simulink model "model_T_PSH_IEEE39"  (R2020b)
settings: Solver=ode3  StartTime=0.0  StopTime=300  FixedStep=Ts  RelTol=1e-3
PostLoadFcn:
  | IEEE39BusLineLength;
  | vNomHV = 345E3;fNom=60;load('Dynamicload.mat');
InitFcn:
  | IEEE39BusLineLength;
  | vNomHV = 345E3;fNom=60;load('Dynamicload.mat');
values from neighbouring files (symbols this model uses):
  At = 1.48    [MAIN_T_PSH_IEEE39.m]
  Dturb = 0.3    [MAIN_T_PSH_IEEE39.m]
  fix_mode = 1    [MAIN_T_PSH_IEEE39.m]
  Gmax = 1    [MAIN_T_PSH_IEEE39.m]
  Gmin = 0    [MAIN_T_PSH_IEEE39.m]
  Hdam = 1    [MAIN_T_PSH_IEEE39.m]
  Kd = 1    [MAIN_T_PSH_IEEE39.m]    (also in plots_T_PSH_IEEE39.m)
  max_delay_gen2pump = 20    [MAIN_T_PSH_IEEE39.m]
  max_delay_pump2hsc = 30    [MAIN_T_PSH_IEEE39.m]
  pgen_pump = Kd*Pref    (= 0.9)    [MAIN_T_PSH_IEEE39.m]
  pgen_turb = (1-Kd)*Pref    (= 0)    [MAIN_T_PSH_IEEE39.m]
  pgen_turb_gen2pump = (1-kd_gen2pump)*Pref    (= 0)    [MAIN_T_PSH_IEEE39.m]
  pgen_turb_hsc2gen = (1-kd_hsc2gen)*Pref    (= 0.36)    [MAIN_T_PSH_IEEE39.m]
  pgen_turb_pump2hsc = (1-kd_pump2hsc)*Pref    (= 0.36)    [MAIN_T_PSH_IEEE39.m]
  Pref = 0.9    [MAIN_T_PSH_IEEE39.m]    (also in MAIN_VS_PSH.m = 1)
  qNL = 0.1    [MAIN_T_PSH_IEEE39.m]
  R = 0.04    [MAIN_T_PSH_IEEE39.m]
  r = 0.31    [MAIN_T_PSH_IEEE39.m]
  Rp = 0.05    [IEEE39BusLineLength.m]
  Sn = 320E6    (= 320000000)    [MAIN_T_PSH_IEEE39.m]
  t_gen2pump = 10    [MAIN_T_PSH_IEEE39.m]
  t_hsc2gen = 150    [MAIN_T_PSH_IEEE39.m]
  t_pump2hsc = 35    [MAIN_T_PSH_IEEE39.m]
  t_sw_off = 220    [MAIN_FS_PSH_IEEE39.m]    (also in MAIN_T_PSH_IEEE39.m; MAIN_VS_PSH.m = 45)
  t_sw_on = 130    [MAIN_FS_PSH_IEEE39.m]    (also in MAIN_T_PSH_IEEE39.m; MAIN_VS_PSH.m = 35)
  Tf = 0.05    [MAIN_T_PSH_IEEE39.m]
  Tg = 0.5    [MAIN_T_PSH_IEEE39.m]
  TL_10_11_len = 14    [IEEE39BusLineLength.m]
  TL_10_13_len = 14    [IEEE39BusLineLength.m]
  TL_13_14_len = 32    [IEEE39BusLineLength.m]
  TL_14_15_len = 70    [IEEE39BusLineLength.m]
  TL_15_16_len = 31.5    [IEEE39BusLineLength.m]
  TL_16_17_len = 26    [IEEE39BusLineLength.m]
  TL_16_19_len = 61    [IEEE39BusLineLength.m]
  TL_16_21_len = 46    [IEEE39BusLineLength.m]
  TL_16_24_len = 15    [IEEE39BusLineLength.m]
  TL_17_18_len = 26    [IEEE39BusLineLength.m]
  TL_17_27_len = 59    [IEEE39BusLineLength.m]
  TL_1_2_len = 134    [IEEE39BusLineLength.m]
  TL_1_39_len = 105    [IEEE39BusLineLength.m]
  TL_21_22_len = 47    [IEEE39BusLineLength.m]
  TL_22_23_len = 33    [IEEE39BusLineLength.m]
  TL_24_23_len = 88    [IEEE39BusLineLength.m]
  TL_25_26_len = 101    [IEEE39BusLineLength.m]
  TL_26_27_len = 46.5    [IEEE39BusLineLength.m]
  TL_26_28_len = 151    [IEEE39BusLineLength.m]
  TL_26_29_len = 200    [IEEE39BusLineLength.m]
  TL_28_29_len = 48    [IEEE39BusLineLength.m]
  TL_2_25_len = 28    [IEEE39BusLineLength.m]
  TL_2_2_len = 49    [IEEE39BusLineLength.m]
  TL_3_18_len = 42    [IEEE39BusLineLength.m]
  TL_3_4_len = 53    [IEEE39BusLineLength.m]
  TL_4_14_len = 33    [IEEE39BusLineLength.m]
  TL_4_5_len = 32.5    [IEEE39BusLineLength.m]
  TL_5_6_len = 14    [IEEE39BusLineLength.m]
  TL_5_8_len = 32    [IEEE39BusLineLength.m]
  TL_6_11_len = 26.5    [IEEE39BusLineLength.m]
  TL_6_7_len = 25.5    [IEEE39BusLineLength.m]
  TL_7_8_len = 15    [IEEE39BusLineLength.m]
  TL_8_9_len = 93    [IEEE39BusLineLength.m]
  TL_9_39_len = 136    [IEEE39BusLineLength.m]
  Tr = 6.88    [MAIN_T_PSH_IEEE39.m]
  Ts = 25e-6    (= 2.5e-05)    [MAIN_FS_PSH_IEEE39.m]    (also in MAIN_T_PSH_IEEE39.m; MAIN_VS_PSH.m = 1e-07)
  Velm = 0.05    [MAIN_T_PSH_IEEE39.m]
  Vn = 18000    [MAIN_T_PSH_IEEE39.m]
undefined symbols (not defined in the file or in its folder): D1, Delta, load15, load16, load18, load20, load21, load23, load24, load25, load26, load27, load28, load29, load3, load39, load4, load7, load8
libraries: powerlib x216, sps_avr x10, simulink_extras x7, powerlib_meascontrol x5, simulink x1
(part 6 of 9)

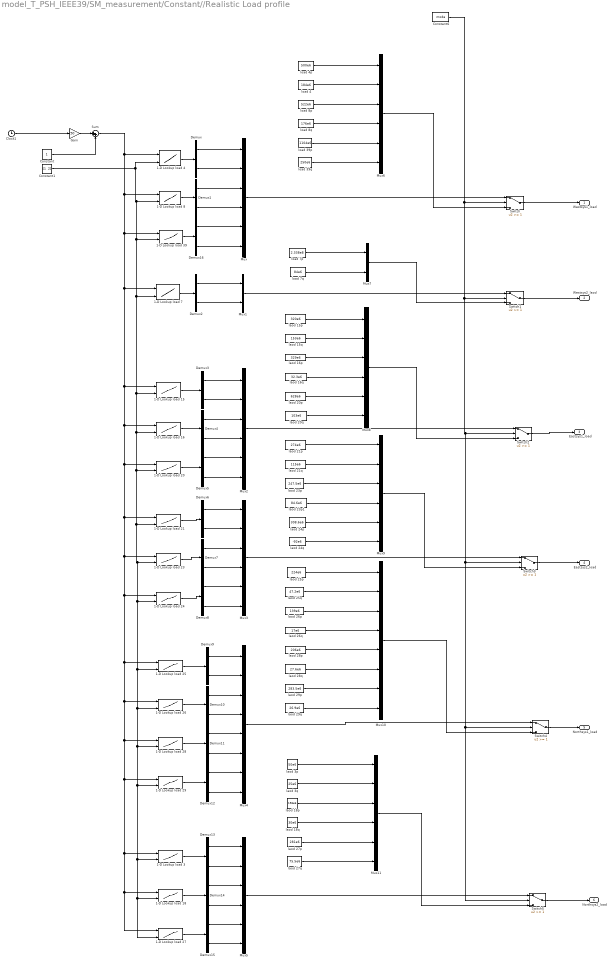
== system model_T_PSH_IEEE39/SM_measurement/Constant//Realistic Load profile ==
  1-D Lookup load 15 : Lookup_n-D  BreakpointsForDimension1=[1:18000]  BreakpointsForDimension2=[1 2]  Table=load15  InterpMethod=Flat  ExtrapMethod=Cubic spline  DiagnosticForOutOfRangeInput=Error  InternalRulePriority=Speed  RndMeth=Simplest  InputSameDT=on
      settings: InputPortMap=u0,u1
  1-D Lookup load 16 : Lookup_n-D  BreakpointsForDimension1=[1:18000]  BreakpointsForDimension2=[1 2]  Table=load16  InterpMethod=Flat  ExtrapMethod=Cubic spline  DiagnosticForOutOfRangeInput=Error  InternalRulePriority=Speed  RndMeth=Simplest  InputSameDT=on
      settings: InputPortMap=u0,u1
  1-D Lookup load 18 : Lookup_n-D  BreakpointsForDimension1=[1:18000]  BreakpointsForDimension2=[1 2]  Table=load18  InterpMethod=Flat  ExtrapMethod=Cubic spline  DiagnosticForOutOfRangeInput=Error  InternalRulePriority=Speed  RndMeth=Simplest  InputSameDT=on
      settings: InputPortMap=u0,u1
  1-D Lookup load 20 : Lookup_n-D  BreakpointsForDimension1=[1:18000]  BreakpointsForDimension2=[1 2]  Table=load20  InterpMethod=Flat  ExtrapMethod=Cubic spline  DiagnosticForOutOfRangeInput=Error  InternalRulePriority=Speed  RndMeth=Simplest  InputSameDT=on
      settings: InputPortMap=u0,u1
  1-D Lookup load 21 : Lookup_n-D  BreakpointsForDimension1=[1:18000]  BreakpointsForDimension2=[1 2]  Table=load21  InterpMethod=Flat  ExtrapMethod=Cubic spline  DiagnosticForOutOfRangeInput=Error  InternalRulePriority=Speed  RndMeth=Simplest  InputSameDT=on
      settings: InputPortMap=u0,u1
  1-D Lookup load 23 : Lookup_n-D  BreakpointsForDimension1=[1:18000]  BreakpointsForDimension2=[1 2]  Table=load23  InterpMethod=Flat  ExtrapMethod=Cubic spline  DiagnosticForOutOfRangeInput=Error  InternalRulePriority=Speed  RndMeth=Simplest  InputSameDT=on
      settings: InputPortMap=u0,u1
  1-D Lookup load 24 : Lookup_n-D  BreakpointsForDimension1=[1:18000]  BreakpointsForDimension2=[1 2]  Table=load24  InterpMethod=Flat  ExtrapMethod=Cubic spline  DiagnosticForOutOfRangeInput=Error  InternalRulePriority=Speed  RndMeth=Simplest  InputSameDT=on
      settings: InputPortMap=u0,u1
  1-D Lookup load 25 : Lookup_n-D  BreakpointsForDimension1=[1:18000]  BreakpointsForDimension2=[1 2]  Table=load25  InterpMethod=Flat  ExtrapMethod=Cubic spline  DiagnosticForOutOfRangeInput=Error  InternalRulePriority=Speed  RndMeth=Simplest  InputSameDT=on
      settings: InputPortMap=u0,u1
  1-D Lookup load 26 : Lookup_n-D  BreakpointsForDimension1=[1:18000]  BreakpointsForDimension2=[1 2]  Table=load26  InterpMethod=Flat  ExtrapMethod=Cubic spline  DiagnosticForOutOfRangeInput=Error  InternalRulePriority=Speed  RndMeth=Simplest  InputSameDT=on
      settings: InputPortMap=u0,u1
  1-D Lookup load 27 : Lookup_n-D  BreakpointsForDimension1=[1:18000]  BreakpointsForDimension2=[1 2]  Table=load27  InterpMethod=Flat  ExtrapMethod=Cubic spline  DiagnosticForOutOfRangeInput=Error  InternalRulePriority=Speed  RndMeth=Simplest  InputSameDT=on
      settings: InputPortMap=u0,u1
  1-D Lookup load 28 : Lookup_n-D  BreakpointsForDimension1=[1:18000]  BreakpointsForDimension2=[1 2]  Table=load28  InterpMethod=Flat  ExtrapMethod=Cubic spline  DiagnosticForOutOfRangeInput=Error  InternalRulePriority=Speed  RndMeth=Simplest  InputSameDT=on
      settings: InputPortMap=u0,u1
  1-D Lookup load 29 : Lookup_n-D  BreakpointsForDimension1=[1:18000]  BreakpointsForDimension2=[1 2]  Table=load29  InterpMethod=Flat  ExtrapMethod=Cubic spline  DiagnosticForOutOfRangeInput=Error  InternalRulePriority=Speed  RndMeth=Simplest  InputSameDT=on
      settings: InputPortMap=u0,u1
  1-D Lookup load 3 : Lookup_n-D  BreakpointsForDimension1=[1:18000]  BreakpointsForDimension2=[1 2]  Table=load3  InterpMethod=Flat  ExtrapMethod=Cubic spline  DiagnosticForOutOfRangeInput=Error  InternalRulePriority=Speed  RndMeth=Simplest  InputSameDT=on
      settings: InputPortMap=u0,u1
  1-D Lookup load 39 : Lookup_n-D  BreakpointsForDimension1=[1:18000]  BreakpointsForDimension2=[1 2]  Table=load39  InterpMethod=Flat  ExtrapMethod=Cubic spline  DiagnosticForOutOfRangeInput=Error  InternalRulePriority=Speed  RndMeth=Simplest  InputSameDT=on
      settings: InputPortMap=u0,u1
  1-D Lookup load 4 : Lookup_n-D  BreakpointsForDimension1=[1:18000]  BreakpointsForDimension2=[1 2]  Table=load4  InterpMethod=Flat  ExtrapMethod=Cubic spline  DiagnosticForOutOfRangeInput=Error  InternalRulePriority=Speed  RndMeth=Simplest  InputSameDT=on
      settings: InputPortMap=u0,u1
  1-D Lookup load 7 : Lookup_n-D  BreakpointsForDimension1=[1:18000]  BreakpointsForDimension2=[1 2]  Table=load7  InterpMethod=Flat  ExtrapMethod=Cubic spline  DiagnosticForOutOfRangeInput=Error  InternalRulePriority=Speed  RndMeth=Simplest  InputSameDT=on
      settings: InputPortMap=u0,u1
  1-D Lookup load 8 : Lookup_n-D  BreakpointsForDimension1=[1:18000]  BreakpointsForDimension2=[1 2]  Table=load8  InterpMethod=Flat  ExtrapMethod=Cubic spline  DiagnosticForOutOfRangeInput=Error  InternalRulePriority=Speed  RndMeth=Simplest  InputSameDT=on
      settings: InputPortMap=u0,u1
  Clock1 : Clock
  Constant : Constant  SampleTime=20e-3
  Constant1 : Constant  Value="[1  2]"  VectorParams1D=off  SampleTime=20e-3
  Constant6 : Constant  Value=mode
  Demux{,1..16} (17 alike) : Demux  Outputs=2
  Gain : Gain  Gain=50
  Mux{,2..3,5..6,8..9,11} (8 alike) : Mux  Inputs=6
  Mux1 : Mux  Inputs=2
  Mux10 : Mux  Inputs=8
  Mux4 : Mux  Inputs=8
  Mux7 : Mux  Inputs=2
  Sum : Sum  Inputs=|++
  Switch{,1..5} (6 alike) : Switch  Threshold=1
  laod 15p : Constant  Value=320e6  VectorParams1D=off  SampleTime=20e-3
  laod 15q : Constant  Value=153e6  VectorParams1D=off  SampleTime=20e-3
  laod 16p : Constant  Value=329e6  VectorParams1D=off  SampleTime=20e-3
  laod 16q : Constant  Value=32.3e6  VectorParams1D=off  SampleTime=20e-3
  laod 18p : Constant  Value=158e6  VectorParams1D=off  SampleTime=20e-3
  laod 18q : Constant  Value=30e6  VectorParams1D=off  SampleTime=20e-3
  laod 20p : Constant  Value=628e6  VectorParams1D=off  SampleTime=20e-3
  laod 20q : Constant  Value=103e6  VectorParams1D=off  SampleTime=20e-3
  laod 21p : Constant  Value=274e6  VectorParams1D=off  SampleTime=20e-3
  laod 21q : Constant  Value=115e6  VectorParams1D=off  SampleTime=20e-3
  laod 23p : Constant  Value=247.5e6  VectorParams1D=off  SampleTime=20e-3
  laod 23p1 : Constant  Value=84.6e6  VectorParams1D=off  SampleTime=20e-3
  laod 24p : Constant  Value=308.6e6  SampleTime=20e-3
  laod 24q : Constant  Value=-92e6  VectorParams1D=off  SampleTime=20e-3
  laod 25p : Constant  Value=224e6  VectorParams1D=off  SampleTime=20e-3
  laod 25q : Constant  Value=47.2e6  VectorParams1D=off  SampleTime=20e-3
  laod 26p : Constant  Value=139e6  VectorParams1D=off  SampleTime=20e-3
  laod 26q : Constant  Value=17e6  VectorParams1D=off  SampleTime=20e-3
  laod 27p : Constant  Value=281e6  VectorParams1D=off  SampleTime=20e-3
  laod 27q : Constant  Value=75.5e6  VectorParams1D=off  SampleTime=20e-3
  laod 28p : Constant  Value=206e6  VectorParams1D=off  SampleTime=20e-3
  laod 28q : Constant  Value=27.6e6  VectorParams1D=off  SampleTime=20e-3
  laod 29p : Constant  Value=283.5e6  VectorParams1D=off  SampleTime=20e-3
  laod 29q : Constant  Value=26.9e6  VectorParams1D=off  SampleTime=20e-3
  laod 3p : Constant  Value=50e6  VectorParams1D=off  SampleTime=20e-3
  laod 3q : Constant  Value=25e6  VectorParams1D=off  SampleTime=20e-3
  load 39p : Constant  Value=1104e6  VectorParams1D=off  SampleTime=20e-3
  load 39q : Constant  Value=250e6  VectorParams1D=off  SampleTime=20e-3
  load 4 : Constant  Value=184e6  VectorParams1D=off  SampleTime=20e-3
  load 4p : Constant  Value=500e6  VectorParams1D=off  SampleTime=20e-3
  load 7p : Constant  Value=2.338e8  VectorParams1D=off  SampleTime=20e-3
  load 7q : Constant  Value=84e6  VectorParams1D=off  SampleTime=20e-3
  load 8p : Constant  Value=522e6  VectorParams1D=off  SampleTime=20e-3
  load 8q : Constant  Value=176e6  VectorParams1D=off  SampleTime=20e-3
  Westsys1_load : Outport
  Westsys2_laod : Outport  Port=2
  Eastsys1_load : Outport  Port=3
  Eastsys2_load : Outport  Port=4
  Northsys1_load : Outport  Port=5
  Northsys2_load : Outport  Port=6
  wires:
  Mux2/1 -> Switch2/1
  Constant/1 -> Sum/2
  Mux/1 -> Switch/1
  Mux1/1 -> Switch1/1
  Mux5/1 -> Switch5/1
  1-D Lookup load 15/1 -> Demux3/1
  Demux2/2 -> Mux1/2
  Demux5/2 -> Mux2/6
  Demux7/2 -> Mux3/4
  Demux10/2 -> Mux4/4
  Sum/1 -> 1-D Lookup load 28/1, 1-D Lookup load 27/1, 1-D Lookup load 18/1, 1-D Lookup load 3/1, 1-D Lookup load 29/1, 1-D Lookup load 26/1, 1-D Lookup load 25/1, 1-D Lookup load 24/1, 1-D Lookup load 23/1, 1-D Lookup load 21/1, 1-D Lookup load 20/1, 1-D Lookup load 16/1, 1-D Lookup load 15/1, 1-D Lookup load 7/1, 1-D Lookup load 39/1, 1-D Lookup load 8/1, 1-D Lookup load 4/1
  1-D Lookup load 4/1 -> Demux/1
  Demux/1 -> Mux/1
  Demux/2 -> Mux/2
  1-D Lookup load 8/1 -> Demux1/1
  Demux1/1 -> Mux/3
  Demux1/2 -> Mux/4
  Demux16/1 -> Mux/5
  Demux16/2 -> Mux/6
  1-D Lookup load 39/1 -> Demux16/1
  1-D Lookup load 7/1 -> Demux2/1
  Demux2/1 -> Mux1/1
  Demux3/1 -> Mux2/1
  Demux3/2 -> Mux2/2
  1-D Lookup load 16/1 -> Demux4/1
  Demux4/1 -> Mux2/3
  Demux4/2 -> Mux2/4
  Demux5/1 -> Mux2/5
  1-D Lookup load 20/1 -> Demux5/1
  Demux6/2 -> Mux3/2
  Demux6/1 -> Mux3/1
  1-D Lookup load 21/1 -> Demux6/1
  Demux7/1 -> Mux3/3
  1-D Lookup load 23/1 -> Demux7/1
  1-D Lookup load 24/1 -> Demux8/1
  Demux8/1 -> Mux3/5
  Demux8/2 -> Mux3/6
  Demux9/2 -> Mux4/2
  Demux9/1 -> Mux4/1
  1-D Lookup load 25/1 -> Demux9/1
  1-D Lookup load 26/1 -> Demux10/1
  Demux10/1 -> Mux4/3
  Demux11/1 -> Mux4/5
  Demux11/2 -> Mux4/6
  1-D Lookup load 28/1 -> Demux11/1
  Demux12/1 -> Mux4/7
  Demux12/2 -> Mux4/8
  1-D Lookup load 29/1 -> Demux12/1
  1-D Lookup load 3/1 -> Demux13/1
  Demux13/1 -> Mux5/1
  Demux13/2 -> Mux5/2
  Constant1/1 -> 1-D Lookup load 7/2, 1-D Lookup load 20/2, 1-D Lookup load 27/2, 1-D Lookup load 18/2, 1-D Lookup load 3/2, 1-D Lookup load 29/2, 1-D Lookup load 28/2, 1-D Lookup load 26/2, 1-D Lookup load 25/2, 1-D Lookup load 24/2, 1-D Lookup load 23/2, 1-D Lookup load 21/2, 1-D Lookup load 16/2, 1-D Lookup load 15/2, 1-D Lookup load 39/2, 1-D Lookup load 8/2, 1-D Lookup load 4/2
  Demux14/1 -> Mux5/3
  Demux14/2 -> Mux5/4
  1-D Lookup load 18/1 -> Demux14/1
  Demux15/1 -> Mux5/5
  Demux15/2 -> Mux5/6
  1-D Lookup load 27/1 -> Demux15/1
  Clock1/1 -> Gain/1
  Gain/1 -> Sum/1
  Mux6/1 -> Switch/3
  load 4p/1 -> Mux6/1
  load 4/1 -> Mux6/2
  load 8p/1 -> Mux6/3
  load 8q/1 -> Mux6/4
  load 39p/1 -> Mux6/5
  load 39q/1 -> Mux6/6
  Constant6/1 -> Switch5/2, Switch4/2, Switch3/2, Switch2/2, Switch1/2, Switch/2
  Switch/1 -> Westsys1_load/1
  Mux7/1 -> Switch1/3
  load 7q/1 -> Mux7/2
  load 7p/1 -> Mux7/1
  Switch1/1 -> Westsys2_laod/1
  Switch2/1 -> Eastsys1_load/1
  laod 20q/1 -> Mux8/6
  laod 15p/1 -> Mux8/1
  laod 15q/1 -> Mux8/2
  laod 16p/1 -> Mux8/3
  laod 16q/1 -> Mux8/4
  laod 20p/1 -> Mux8/5
  Mux8/1 -> Switch2/3
  Switch3/1 -> Eastsys2_load/1
  Mux3/1 -> Switch3/1
  laod 23p1/1 -> Mux9/4
  laod 21q/1 -> Mux9/2
  laod 21p/1 -> Mux9/1
  laod 23p/1 -> Mux9/3
  laod 24p/1 -> Mux9/5
  laod 24q/1 -> Mux9/6
  Mux9/1 -> Switch3/3
  Mux10/1 -> Switch4/3
  laod 26q/1 -> Mux10/4
  laod 25q/1 -> Mux10/2
  laod 25p/1 -> Mux10/1
  laod 26p/1 -> Mux10/3
  laod 28p/1 -> Mux10/5
  laod 28q/1 -> Mux10/6
  laod 29p/1 -> Mux10/7
  laod 29q/1 -> Mux10/8
  Switch4/1 -> Northsys1_load/1
  Mux4/1 -> Switch4/1
  Mux11/1 -> Switch5/3
  laod 3p/1 -> Mux11/1
  laod 3q/1 -> Mux11/2
  laod 18p/1 -> Mux11/3
  laod 18q/1 -> Mux11/4
  laod 27p/1 -> Mux11/5
  laod 27q/1 -> Mux11/6
  Switch5/1 -> Northsys2_load/1

== system model_T_PSH_IEEE39/SM_measurement/GT control ==
  note: 10
  note: 9
  note: 8
  note: 7
  note: 6
  note: 5
  note: 4
  note: 3
  note: 2
  note: 1
  Bus Creator : BusCreator  Inputs=3
  Constant{1..6,8,10,12,14} (10 alike) : Constant
  Mux1 : Mux  Inputs=3
  Mux2 : Mux
  Mux6 : Mux  Inputs=3
  GT_CBs_ctrl : Outport
  wires:
  Constant1/1 -> Mux1/2
  Constant10/1 -> Mux1/1
  Constant12/1 -> Mux2/4
  Constant5/1 -> Mux2/3
  Constant2/1 -> Mux2/2
  Constant3/1 -> Mux2/1
  Constant4/1 -> Mux6/3
  Constant8/1 -> Mux6/2
  Constant14/1 -> Mux1/3
  Constant6/1 -> Mux6/1
  Bus Creator/1 -> GT_CBs_ctrl/1
  Mux2/1 -> Bus Creator/2  "Eastsystem GT ctrl"
  Mux6/1 -> Bus Creator/1  "Westsystem GT ctrl"
  Mux1/1 -> Bus Creator/3  "Northsystem GT ctrl"

== system model_T_PSH_IEEE39/SS_EastSystem1/Buses current_E ==
  Mux3 : Mux  Inputs=5
  current : Outport
  wires:
  Mux3/1 -> current/1
  [I_bus_14] -> Mux3/1
  [I_L15] -> Mux3/2
  [I_L16] -> Mux3/3
  [I_bus_19] -> Mux3/4
  [I_L20] -> Mux3/5

== system model_T_PSH_IEEE39/SS_EastSystem1/Buses voltages_E ==
  Mux3 : Mux  Inputs=5
  Voltages : Outport
  wires:
  [V_L20] -> Mux3/5
  [V_bus_19] -> Mux3/4
  [V_L16] -> Mux3/3
  [V_L15] -> Mux3/2
  [V_bus_14] -> Mux3/1
  Mux3/1 -> Voltages/1

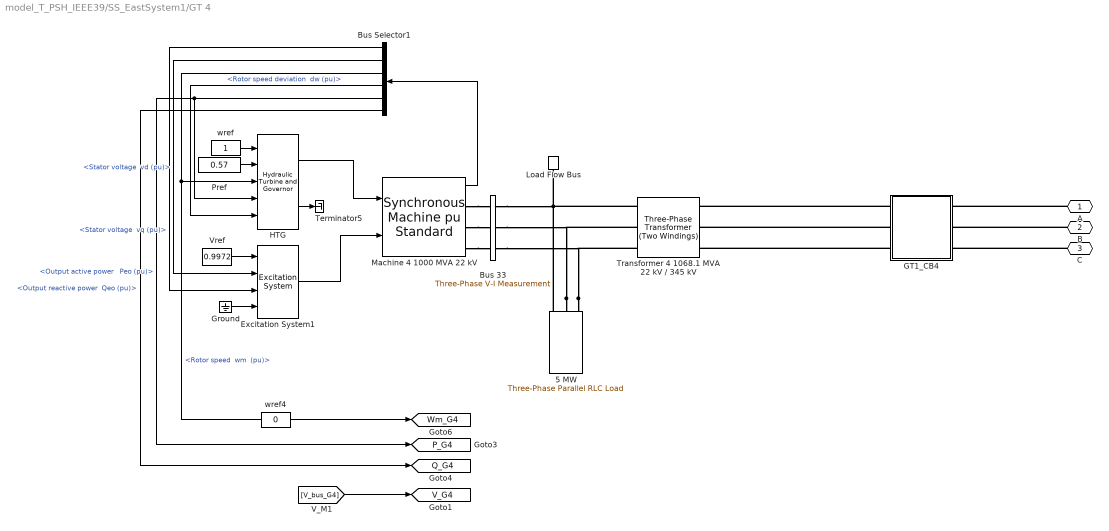
== system model_T_PSH_IEEE39/SS_EastSystem1/GT 4 ==
  5 MW : powerlib/Elements/Three-Phase Parallel RLC Load  LConnTagsString=A|B|C  Configuration=Y (grounded)  NominalVoltage=22e3  Vabc=[1e3 1e3 1e3]  Vabcp=[1e3 1e3 1e3]  NominalFrequency=fNom  UnbalancedPower=off  ActivePower=5e6  InductivePower=0  CapacitivePower=0  Pabc=[10e3 9e3 11e3]  QLabc=[100 90 110]  QCabc=[100 90 110]  Pabcp=[10e3 9e3 11e3]  QLabcp=[100 90 110]  QCabcp=[100 90 110]  Measurements=None  LoadType=constant Z
  Bus Selector1 : BusSelector  OutputSignals="dq0 components.Stator voltage  vq (pu),dq0 components.Stator voltage  vd (pu),Mechanical.Rotor speed  wm  (pu),Mechanical.Rotor speed deviation  dw (pu),Output active power   Peo (pu),Output reactive power  Qeo (pu)"
  Bus 33 : powerlib/Measurements/Three-Phase V-I Measurement  VoltageMeasurement=phase-to-ground  SetLabelV=on  LabelV=V_bus_G4  Vpu=off  VpuLL=off  CurrentMeasurement=no  SetLabelI=on  LabelI=I_bus_G4  Ipu=off  Pbase=100e6  Vbase=16.5e3  OutputType=Complex  PhasorSimulation=off  PSBequivalent=0
  Excitation System1 : sps_avr/Excitation System  tr=20e-3  reg=[ 200, 0.02 ]  exc=[ 1, 0 .19]  tgr=[ 0, 0 ]  damp=[ 0.0012, 1 ]  sat=[ 0, 0 ]  lim=[ 0, 7.32, 0 ]  v0=[0.9972 1.7419]
      settings: SourceProductBaseCode=PS
  GT1_CB4 : Subsystem
  Ground : Ground
  HTG : powerlib/Machines/Hydraulic Turbine and Governor  sm="[ 10/3  0.07 ]"  gate="[  0.01  0.97518  -0.1  0.1 ]"  reg="[ Rp  1.163  0.105  0  0.01  ]"  hyd="[  0  2.67  ]"  dref=0  po=0.57
      settings: SourceProductBaseCode=PS
  Load Flow Bus : powerlib/Measurements/Load Flow Bus  LConnTagsString=a  Phases=single  Connectors=on one side  ID=Bus-33  Vbase=22000  Vref=0.9972  Vangle=0  VLF=0.9972  VLFb=1  VLFc=1  angleLF=-4.252  angleLFb=0  angleLFc=0
      settings: AttributesFormatString=%<ID>\n%<Vbase>V\n%<VLF>pu\n%<angleLF>deg.
  Machine 4 1000 MVA 22 kV : powerlib/Machines/Synchronous Machine pu Standard  PresetModel=No  MechanicalLoad=Mechanical power Pm  ShowDetailedParameters=on  RotorType=Round  Units=per unit standard parameters  MeasurementBus=off  NominalParameters="[ 1000E6  22000   fNom]"  Reactances1="[ 2.403 0.4 0.2 2.367 1.523 0.2 0.03  ]"  Reactances2=[ 0.995, 0.195, 0.155, 0.568, 0.143, 0.16 ]  dAxisTimeConstants=Open-circuit  qAxisTimeConstants=Open-circuit  TimeConstants1=[]  TimeConstants2=[5.69 0.03 1.5 0.04]  TimeConstants3=[]  TimeConstants4=[]  TimeConstants5=[ 9.2, 0.01, 0.01 ]  TimeConstants6=[]  TimeConstants7=[]  TimeConstants8=[]  StatorResistance=0.005  Mechanical=[ 3.117 0.02 20]  PolePairs=20  InitialConditions=[0 -47.2467 0.538718 0.538718 0.538718 -12.2371 -132.237 107.763 1.74187]  SetSaturation=off  Saturation=[0.6404,0.7127,0.8441,0.9214,0.9956,1.082,1.19,1.316,1.457;0.7,0.7698,0.8872,0.9466,0.9969,1.046,1.1,1.151,1.201]  LoadFlowParameters=[1 632000000 21938.4 0]  TsPowergui=0  TsBlock=-1  IterativeModel=Trapezoidal non iterative  IterativeDiscreteModel=Trapezoidal non iterative  BusType=PV  Pref=5.32e+008  Qref=0  Qmin=-500e6  Qmax=150e6  PLF=0  QLF=0
      settings: AttributesFormatString=\n\n
  Pref : Constant  Value=0.57
  Terminator5 : Terminator
  Transformer 4 1068.1 MVA 22 kV / 345 kV : powerlib/Elements/Three-Phase Transformer (Two Windings)  Winding1Connection=Delta (D1)  Winding2Connection=Yg  CoreType=Three single-phase transformers  SetSaturation=off  Hysteresis=off  DataFile='hysteresis'  SetInitialFlux=off  Measurements=None  UNITS=pu  NominalPower=[ 1068.1e6 fNom]  Winding1="[ 22e3 0.007*1068.1/100/2      0.0142*1068.1/100/2 ]"  Winding2="[ 1.07*345e3 0.007*1068.1/100/2      0.0142*1068.1/100/2]"  Rm=500  Lm=500  L0=0.5  Saturation="[ 0,0  ;  0.005,1.2  ;  1.0,1.4 ]"  InitialFluxes=[ 0.8 , -0.8 , 0.7 ]  BreakLoop=off  DiscreteSolver=Trapezoidal iterative  DataType=off  TransfoNumber=0
  Vref : Constant  Value=0.9972
  wref : Constant
  wref4 : Constant  Value=0
  A : PMIOPort  Side=Right
  B : PMIOPort  Port=2  Side=Right
  C : PMIOPort  Port=3  Side=Right
  tag scope: P_G4=global, Q_G4=global, V_G4=global, Wm_G4=global
  wires:
  [V_bus_G4] -> [V_G4]
  Bus Selector1/6 -> [Q_G4]  "<Output reactive power  Qeo (pu)>"
  Bus Selector1/5 -> [P_G4], HTG/4  "<Output active power   Peo (pu)>"
  Bus Selector1/4 -> HTG/5  "<Rotor speed deviation  dw (pu)>"
  Bus Selector1/3 -> [Wm_G4], HTG/3  "<Rotor speed  wm  (pu)>"
  Bus Selector1/2 -> Excitation System1/2  "<Stator voltage  vd (pu)>"
  Bus Selector1/1 -> Excitation System1/3  "<Stator voltage  vq (pu)>"
  Machine 4 1000 MVA 22 kV/1 -> Bus Selector1/1
  Excitation System1/1 -> Machine 4 1000 MVA 22 kV/2
  wref/1 -> HTG/1
  Pref/1 -> HTG/2
  Vref/1 -> Excitation System1/1
  HTG/2 -> Terminator5/1
  Ground/1 -> Excitation System1/4
  HTG/1 -> Machine 4 1000 MVA 22 kV/1
  connections:
  Machine 4 1000 MVA 22 kV/RConn3 -- Bus 33/LConn3
  Machine 4 1000 MVA 22 kV/RConn2 -- Bus 33/LConn2
  Machine 4 1000 MVA 22 kV/RConn1 -- Bus 33/LConn1
  5 MW/LConn3 -- Bus 33/RConn3 -- Transformer 4 1068.1 MVA 22 kV / 345 kV/LConn3
  5 MW/LConn2 -- Bus 33/RConn2 -- Transformer 4 1068.1 MVA 22 kV / 345 kV/LConn2
  5 MW/LConn1 -- Bus 33/RConn1 -- Load Flow Bus/LConn1 -- Transformer 4 1068.1 MVA 22 kV / 345 kV/LConn1
  GT1_CB4/LConn1 -- Transformer 4 1068.1 MVA 22 kV / 345 kV/RConn1
  GT1_CB4/LConn2 -- Transformer 4 1068.1 MVA 22 kV / 345 kV/RConn2
  GT1_CB4/LConn3 -- Transformer 4 1068.1 MVA 22 kV / 345 kV/RConn3
  C/RConn1 -- GT1_CB4/RConn3
  B/RConn1 -- GT1_CB4/RConn2
  A/RConn1 -- GT1_CB4/RConn1

== system model_T_PSH_IEEE39/SS_EastSystem1/GT 5 ==
  5 MW : powerlib/Elements/Three-Phase Parallel RLC Load  LConnTagsString=A|B|C  Configuration=Y (grounded)  NominalVoltage=22e3  Vabc=[1e3 1e3 1e3]  Vabcp=[1e3 1e3 1e3]  NominalFrequency=fNom  UnbalancedPower=off  ActivePower=5e6  InductivePower=0  CapacitivePower=0  Pabc=[10e3 9e3 11e3]  QLabc=[100 90 110]  QCabc=[100 90 110]  Pabcp=[10e3 9e3 11e3]  QLabcp=[100 90 110]  QCabcp=[100 90 110]  Measurements=None  LoadType=constant Z
  Bus Selector1 : BusSelector  OutputSignals="dq0 components.Stator voltage  vq (pu),dq0 components.Stator voltage  vd (pu),Mechanical.Rotor speed  wm  (pu),Mechanical.Rotor speed deviation  dw (pu),Output active power   Peo (pu),Output reactive power  Qeo (pu)"
  Bus 34 : powerlib/Measurements/Three-Phase V-I Measurement  VoltageMeasurement=phase-to-ground  SetLabelV=on  LabelV=V_bus_G5  Vpu=off  VpuLL=off  CurrentMeasurement=no  SetLabelI=on  LabelI=I_bus_G5  Ipu=off  Pbase=100e6  Vbase=16.5e3  OutputType=Complex  PhasorSimulation=off  PSBequivalent=0
  Excitation System1 : sps_avr/Excitation System  tr=20e-3  reg=[ 200, 0.02 ]  exc=[ 1, 0 .19]  tgr=[ 0, 0 ]  damp=[ 0.0012, 1 ]  sat=[ 0, 0 ]  lim=[ 0, 7.32, 0 ]  v0=[1.0123 3.3412]
      settings: SourceProductBaseCode=PS
  GT1_CB6 : Subsystem
  Ground : Ground
  HTG : powerlib/Machines/Hydraulic Turbine and Governor  sm="[ 10/3  0.07 ]"  gate="[  0.01  0.97518  -0.1  0.1 ]"  reg="[  Rp  1.163  0.105  0  0.01  ]"  hyd="[  0  2.67  ]"  dref=0  po=0.709
      settings: SourceProductBaseCode=PS
  Load Flow Bus : powerlib/Measurements/Load Flow Bus  LConnTagsString=a  Phases=single  Connectors=on one side  ID=Bus-34  Vbase=22000  Vref=1.0123  Vangle=0  VLF=1.012  VLFb=1  VLFc=1  angleLF=-37.01  angleLFb=0  angleLFc=0
      settings: AttributesFormatString=%<ID>\n%<Vbase>V\n%<VLF>pu\n%<angleLF>deg.
  Machine 5 520 MVA 22 kV : powerlib/Machines/Synchronous Machine pu Standard  PresetModel=No  MechanicalLoad=Mechanical power Pm  ShowDetailedParameters=on  RotorType=Round  Units=per unit standard parameters  MeasurementBus=off  NominalParameters="[ 520E6  22000   fNom]"  Reactances1=[ 3.484 0.686 0.343 3.224 0.8632 0.343 0.054 ]  Reactances2=[ 0.995, 0.195, 0.155, 0.568, 0.143, 0.16 ]  dAxisTimeConstants=Open-circuit  qAxisTimeConstants=Open-circuit  TimeConstants1=[]  TimeConstants2=[5.4 0.03 0.44 0.04]  TimeConstants3=[]  TimeConstants4=[]  TimeConstants5=[ 9.2, 0.01, 0.01 ]  TimeConstants6=[]  TimeConstants7=[]  TimeConstants8=[]  StatorResistance=0  Mechanical=[ 5 0.02 20]  PolePairs=20  InitialConditions=[0 -74.2196 0.822255 0.822255 0.822255 -56.5136 -176.514 63.4864 3.34118]  SetSaturation=off  Saturation=[0.6404,0.7127,0.8441,0.9214,0.9956,1.082,1.19,1.316,1.457;0.7,0.7698,0.8872,0.9466,0.9969,1.046,1.1,1.151,1.201]  LoadFlowParameters=[1 508000000 22270.6 0]  TsPowergui=0  TsBlock=-1  IterativeModel=Trapezoidal non iterative  IterativeDiscreteModel=Trapezoidal non iterative  BusType=PV  Pref=4.08e+008  Qref=0  Qmin=-300e6  Qmax=200e6  PLF=0  QLF=0
      settings: AttributesFormatString=\n\n
  Pref : Constant  Value=0.709
  Terminator5 : Terminator
  Transformer 5 572 MVA 22 kV / 345 kV : powerlib/Elements/Three-Phase Transformer (Two Windings)  Winding1Connection=Delta (D1)  Winding2Connection=Yg  CoreType=Three single-phase transformers  SetSaturation=off  Hysteresis=off  DataFile='hysteresis'  SetInitialFlux=off  Measurements=None  UNITS=pu  NominalPower=[ 572e6 fNom]  Winding1="[ 22e3 0.009*572/100/2    0.018*572/100/2]"  Winding2="[ 1.009*345e3 0.009*572/100/2    0.018*572/100/2]"  Rm=500  Lm=500  L0=0.5  Saturation="[ 0,0  ;  0.005,1.2  ;  1.0,1.4 ]"  InitialFluxes=[ 0.8 , -0.8 , 0.7 ]  BreakLoop=off  DiscreteSolver=Trapezoidal iterative  DataType=off  TransfoNumber=0
  Vref : Constant  Value=1.0123
  wref : Constant
  A : PMIOPort  Side=Right
  B : PMIOPort  Port=2  Side=Right
  C : PMIOPort  Port=3  Side=Right
  tag scope: P_G5=global, Q_G5=global, V_G5=global, Wm_G5=global
  wires:
  Ground/1 -> Excitation System1/4
  HTG/2 -> Terminator5/1
  Vref/1 -> Excitation System1/1
  Pref/1 -> HTG/2
  wref/1 -> HTG/1
  HTG/1 -> Machine 5 520 MVA 22 kV/1
  Machine 5 520 MVA 22 kV/1 -> Bus Selector1/1
  Bus Selector1/1 -> Excitation System1/3  "<Stator voltage  vq (pu)>"
  Bus Selector1/2 -> Excitation System1/2  "<Stator voltage  vd (pu)>"
  Bus Selector1/3 -> HTG/3, [Wm_G5]  "<Rotor speed  wm  (pu)>"
  Bus Selector1/4 -> HTG/5  "<Rotor speed deviation  dw (pu)>"
  Bus Selector1/5 -> HTG/4, [P_G5]  "<Output active power   Peo (pu)>"
  Bus Selector1/6 -> [Q_G5]  "<Output reactive power  Qeo (pu)>"
  [V_bus_G5] -> [V_G5]
  Excitation System1/1 -> Machine 5 520 MVA 22 kV/2
  connections:
  Transformer 5 572 MVA 22 kV / 345 kV/LConn1 -- Load Flow Bus/LConn1 -- Bus 34/RConn1 -- 5 MW/LConn1
  Transformer 5 572 MVA 22 kV / 345 kV/LConn2 -- Bus 34/RConn2 -- 5 MW/LConn2
  Transformer 5 572 MVA 22 kV / 345 kV/LConn3 -- Bus 34/RConn3 -- 5 MW/LConn3
  Machine 5 520 MVA 22 kV/RConn1 -- Bus 34/LConn1
  Machine 5 520 MVA 22 kV/RConn2 -- Bus 34/LConn2
  Machine 5 520 MVA 22 kV/RConn3 -- Bus 34/LConn3
  GT1_CB6/LConn1 -- Transformer 5 572 MVA 22 kV / 345 kV/RConn1
  GT1_CB6/LConn2 -- Transformer 5 572 MVA 22 kV / 345 kV/RConn2
  GT1_CB6/LConn3 -- Transformer 5 572 MVA 22 kV / 345 kV/RConn3
  B/RConn1 -- GT1_CB6/RConn2
  A/RConn1 -- GT1_CB6/RConn1
  C/RConn1 -- GT1_CB6/RConn3

== system model_T_PSH_IEEE39/SS_EastSystem1/Load 15 ==
  Bus_L15 : powerlib/Measurements/Three-Phase V-I Measurement  VoltageMeasurement=phase-to-ground  SetLabelV=off  LabelV=V_Bus_L15  Vpu=off  VpuLL=off  CurrentMeasurement=yes  SetLabelI=on  LabelI=I_L15  Ipu=off  Pbase=100e6  Vbase=230e3  OutputType=Complex  PhasorSimulation=off  PSBequivalent=0
  Terminator : Terminator
  Three-Phase Dynamic Load : powerlib/Elements/Three-Phase Dynamic Load  NominalVoltage=[345e3 fNom]  ActiveReactivePowers=[3.2e+08 1.53e+08]  PositiveSequence=[0.99604 18.5295]  ExternalControl=on  NpNq=[0 0]  TimeConstants="[0  0  0  0]"  MinimumVoltage=0.7  Tfilter=1e-4  LoadFlowParameters=[4,0,0,0,0]
      settings: SourceProductBaseCode=PS
  A : PMIOPort  Side=Left
  B : PMIOPort  Port=2  Side=Left
  C : PMIOPort  Port=3  Side=Left
  tag scope: V_L15=global
  wires:
  Three-Phase Dynamic Load/1 -> Terminator/1
  Bus_L15/1 -> [V_L15]
  [load15] -> Three-Phase Dynamic Load/1
  connections:
  C/RConn1 -- Bus_L15/LConn3
  Bus_L15/RConn3 -- Three-Phase Dynamic Load/LConn3
  Bus_L15/RConn2 -- Three-Phase Dynamic Load/LConn2
  A/RConn1 -- Bus_L15/LConn1
  B/RConn1 -- Bus_L15/LConn2
  Bus_L15/RConn1 -- Three-Phase Dynamic Load/LConn1

== system model_T_PSH_IEEE39/SS_EastSystem1/Load 16 ==
  Bus_L16 : powerlib/Measurements/Three-Phase V-I Measurement  VoltageMeasurement=phase-to-ground  SetLabelV=off  LabelV=V_Bus_L16  Vpu=off  VpuLL=off  CurrentMeasurement=yes  SetLabelI=on  LabelI=I_L16  Ipu=off  Pbase=100e6  Vbase=230e3  OutputType=Complex  PhasorSimulation=off  PSBequivalent=0
  Terminator : Terminator
  Three-Phase Dynamic Load : powerlib/Elements/Three-Phase Dynamic Load  NominalVoltage=[345e3 fNom]  ActiveReactivePowers=[3.29e+08 3.23e+07]  PositiveSequence=[1.00736 19.2229]  ExternalControl=on  NpNq=[0 0]  TimeConstants="[0  0  0  0]"  MinimumVoltage=0.7  Tfilter=1e-4  LoadFlowParameters=[4,0,0,0,0]
      settings: SourceProductBaseCode=PS
  A : PMIOPort  Side=Left
  B : PMIOPort  Port=2  Side=Left
  C : PMIOPort  Port=3  Side=Left
  tag scope: V_L16=global
  wires:
  Three-Phase Dynamic Load/1 -> Terminator/1
  Bus_L16/1 -> [V_L16]
  [load16] -> Three-Phase Dynamic Load/1
  connections:
  Three-Phase Dynamic Load/LConn1 -- Bus_L16/RConn1
  C/RConn1 -- Bus_L16/LConn3
  B/RConn1 -- Bus_L16/LConn2
  A/RConn1 -- Bus_L16/LConn1
  Bus_L16/RConn2 -- Three-Phase Dynamic Load/LConn2
  Bus_L16/RConn3 -- Three-Phase Dynamic Load/LConn3

== system model_T_PSH_IEEE39/SS_EastSystem1/Load 20 ==
  Bus_L20 : powerlib/Measurements/Three-Phase V-I Measurement  VoltageMeasurement=phase-to-ground  SetLabelV=off  LabelV=V_Bus_L20  Vpu=off  VpuLL=off  CurrentMeasurement=yes  SetLabelI=on  LabelI=I_L20  Ipu=off  Pbase=100e6  Vbase=230e3  OutputType=Complex  PhasorSimulation=off  PSBequivalent=0
  Snubber : powerlib/Elements/Three-Phase Series RLC Load  LConnTagsString=A|B|C  Configuration=Y (grounded)  NominalVoltage=345E3  Vabc=[1e3 1e3 1e3]  Vabcp=[1e3 1e3 1e3]  NominalFrequency=fNom  UnbalancedPower=off  ActivePower=1e6  InductivePower=0  CapacitivePower=1e7  Pabc=[10e3 9e3 11e3]  QLabc=[100 90 110]  QCabc=[100 90 110]  Pabcp=[10e3 9e3 11e3]  QLabcp=[100 90 110]  QCabcp=[100 90 110]  Measurements=None  LoadType=constant Z
  Terminator : Terminator
  Three-Phase Dynamic Load : powerlib/Elements/Three-Phase Dynamic Load  NominalVoltage=[345e3 fNom]  ActiveReactivePowers=[6.28e+08 1.03e+08]  PositiveSequence=[0.961329 -10.5466]  ExternalControl=on  NpNq=[0 0]  TimeConstants="[0  0  0  0]"  MinimumVoltage=0.7  Tfilter=1e-4  LoadFlowParameters=[4,0,0,0,0]
      settings: SourceProductBaseCode=PS
  A : PMIOPort  Side=Left
  B : PMIOPort  Port=2  Side=Left
  C : PMIOPort  Port=3  Side=Left
  tag scope: V_L20=global
  wires:
  Three-Phase Dynamic Load/1 -> Terminator/1
  Bus_L20/1 -> [V_L20]
  [load20] -> Three-Phase Dynamic Load/1
  connections:
  Bus_L20/RConn3 -- Snubber/LConn3 -- Three-Phase Dynamic Load/LConn3
  Bus_L20/RConn2 -- Snubber/LConn2 -- Three-Phase Dynamic Load/LConn2
  A/RConn1 -- Bus_L20/LConn1
  B/RConn1 -- Bus_L20/LConn2
  C/RConn1 -- Bus_L20/LConn3
  Bus_L20/RConn1 -- Snubber/LConn1 -- Three-Phase Dynamic Load/LConn1

== system model_T_PSH_IEEE39/SS_EastSystem1/Machines Measurements ==
  Mux : Mux  Inputs=2
  Mux1 : Mux
  Mux2 : Mux
  Machines Measurements : Outport
  wires:
  Mux2/1 -> Mux/2
  Mux1/1 -> Mux/1
  Mux/1 -> Machines Measurements/1
  [Wm_G5] -> Mux2/4
  [Q_G5] -> Mux2/3
  [P_G5] -> Mux2/2
  [V_G5] -> Mux2/1
  [Wm_G4] -> Mux1/4
  [Q_G4] -> Mux1/3
  [P_G4] -> Mux1/2
  [V_G4] -> Mux1/1

== system model_T_PSH_IEEE39/SS_EastSystem2/Buses current_E ==
  Mux3 : Mux
  current : Outport
  wires:
  Mux3/1 -> current/1
  [I_L21] -> Mux3/1
  [I_bus_22] -> Mux3/2
  [I_L23] -> Mux3/3
  [I_L24] -> Mux3/4

== system model_T_PSH_IEEE39/SS_EastSystem2/Buses voltages_E ==
  Mux3 : Mux
  Voltages : Outport
  wires:
  [V_L24] -> Mux3/4
  [V_L23] -> Mux3/3
  [V_bus_22] -> Mux3/2
  [V_L21] -> Mux3/1
  Mux3/1 -> Voltages/1

== system model_T_PSH_IEEE39/SS_EastSystem2/GT 6 ==
  5 MW : powerlib/Elements/Three-Phase Parallel RLC Load  LConnTagsString=A|B|C  Configuration=Y (grounded)  NominalVoltage=22e3  Vabc=[1e3 1e3 1e3]  Vabcp=[1e3 1e3 1e3]  NominalFrequency=fNom  UnbalancedPower=off  ActivePower=5e6  InductivePower=0  CapacitivePower=0  Pabc=[10e3 9e3 11e3]  QLabc=[100 90 110]  QCabc=[100 90 110]  Pabcp=[10e3 9e3 11e3]  QLabcp=[100 90 110]  QCabcp=[100 90 110]  Measurements=None  LoadType=constant Z
  Bus Selector1 : BusSelector  OutputSignals="dq0 components.Stator voltage  vq (pu),dq0 components.Stator voltage  vd (pu),Mechanical.Rotor speed  wm  (pu),Mechanical.Rotor speed deviation  dw (pu),Output active power   Peo (pu),Output reactive power  Qeo (pu)"
  Bus 35 : powerlib/Measurements/Three-Phase V-I Measurement  VoltageMeasurement=phase-to-ground  SetLabelV=on  LabelV=V_bus_G6  Vpu=off  VpuLL=off  CurrentMeasurement=no  SetLabelI=on  LabelI=I_bus_G6  Ipu=off  Pbase=100e6  Vbase=16.5e3  OutputType=Complex  PhasorSimulation=off  PSBequivalent=0
  Excitation System : sps_avr/Excitation System  tr=20e-3  reg=[ 200, 0.02 ]  exc=[ 1, 0 .19]  tgr=[ 0, 0 ]  damp=[ 0.0012, 1 ]  sat=[ 0, 0 ]  lim=[ 0, 7.32, 0 ]  v0=[1.02 1.8033]
      settings: SourceProductBaseCode=PS
  GT1_CB8 : Subsystem
  Ground : Ground
  HTG : powerlib/Machines/Hydraulic Turbine and Governor  sm="[ 10/3  0.07 ]"  gate="[  0.01  0.97518  -0.1  0.1 ]"  reg="[  Rp  1.163  0.105  0  0.01  ]"  hyd="[  0  2.67  ]"  dref=0  po=0.51
      settings: SourceProductBaseCode=PS
  Load Flow Bus : powerlib/Measurements/Load Flow Bus  LConnTagsString=a  Phases=single  Connectors=on one side  ID=Bus-35  Vbase=22000  Vref=1.02  Vangle=0  VLF=1.02  VLFb=1  VLFc=1  angleLF=-1.943  angleLFb=0  angleLFc=0
      settings: AttributesFormatString=%<ID>\n%<Vbase>V\n%<VLF>pu\n%<angleLF>deg.
  Machine 6 1000 MVA 22 kV : powerlib/Machines/Synchronous Machine pu Standard  PresetModel=No  MechanicalLoad=Mechanical power Pm  ShowDetailedParameters=on  RotorType=Round  Units=per unit standard parameters  MeasurementBus=off  NominalParameters="[ 1000E6  22000   fNom]"  Reactances1=[ 2.032 0.4 0.2 1.928 0.651 0.2 0.022 ]  Reactances2=[ 0.995, 0.195, 0.155, 0.568, 0.143, 0.16 ]  dAxisTimeConstants=Open-circuit  qAxisTimeConstants=Open-circuit  TimeConstants1=[]  TimeConstants2=[7.3 0.03 0.4 0.04]  TimeConstants3=[]  TimeConstants4=[]  TimeConstants5=[ 9.2, 0.01, 0.01 ]  TimeConstants6=[]  TimeConstants7=[]  TimeConstants8=[]  StatorResistance=0.005  Mechanical=[ 4.35 0.02 20]  PolePairs=20  InitialConditions=[0 -55.6147 0.575854 0.575854 0.575854 -22.492 -142.492 97.508 1.80331]  SetSaturation=off  Saturation=[0.6404,0.7127,0.8441,0.9214,0.9956,1.082,1.19,1.316,1.457;0.7,0.7698,0.8872,0.9466,0.9969,1.046,1.1,1.151,1.201]  LoadFlowParameters=[1 650000000 23084.6 0]  TsPowergui=0  TsBlock=-1  IterativeModel=Trapezoidal non iterative  IterativeDiscreteModel=Trapezoidal non iterative  BusType=PV  Pref=5.50e+008  Qref=0  Qmin=-500e6  Qmax=250e6  PLF=0  QLF=0
      settings: AttributesFormatString=\n\n
  Pref : Constant  Value=0.51
  Terminator5 : Terminator
  Transformer 6 880 MVA 22  kV / 345 kV : powerlib/Elements/Three-Phase Transformer (Two Windings)  Winding1Connection=Delta (D1)  Winding2Connection=Yg  CoreType=Three single-phase transformers  SetSaturation=off  Hysteresis=off  DataFile='hysteresis'  SetInitialFlux=off  Measurements=None  UNITS=pu  NominalPower=[ 880e6 fNom]  Winding1="[ 22e3  0.0   0.0143*880/100/2]"  Winding2="[ 1.025*345e3 0.0   0.0143*880/100/2]"  Rm=500  Lm=500  L0=0.5  Saturation="[ 0,0  ;  0.005,1.2  ;  1.0,1.4 ]"  InitialFluxes=[ 0.8 , -0.8 , 0.7 ]  BreakLoop=off  DiscreteSolver=Trapezoidal iterative  DataType=off  TransfoNumber=0
  Vref : Constant  Value=1.02
  wref : Constant
  A : PMIOPort  Side=Right
  B : PMIOPort  Port=2  Side=Right
  C : PMIOPort  Port=3  Side=Right
  tag scope: P_G6=global, Q_G6=global, V_G6=global, Wm_G6=global
  wires:
  Ground/1 -> Excitation System/4
  HTG/2 -> Terminator5/1
  Vref/1 -> Excitation System/1
  Pref/1 -> HTG/2
  wref/1 -> HTG/1
  Excitation System/1 -> Machine 6 1000 MVA 22 kV/2
  HTG/1 -> Machine 6 1000 MVA 22 kV/1
  Machine 6 1000 MVA 22 kV/1 -> Bus Selector1/1
  Bus Selector1/1 -> Excitation System/3  "<Stator voltage  vq (pu)>"
  Bus Selector1/2 -> Excitation System/2  "<Stator voltage  vd (pu)>"
  Bus Selector1/3 -> HTG/3, [Wm_G6]  "<Rotor speed  wm  (pu)>"
  Bus Selector1/4 -> HTG/5  "<Rotor speed deviation  dw (pu)>"
  Bus Selector1/5 -> HTG/4, [P_G6]  "<Output active power   Peo (pu)>"
  Bus Selector1/6 -> [Q_G6]  "<Output reactive power  Qeo (pu)>"
  [V_bus_G6] -> [V_G6]
  connections:
  Transformer 6 880 MVA 22  kV / 345 kV/LConn1 -- Load Flow Bus/LConn1 -- Bus 35/RConn1 -- 5 MW/LConn1
  Transformer 6 880 MVA 22  kV / 345 kV/LConn2 -- Bus 35/RConn2 -- 5 MW/LConn2
  Transformer 6 880 MVA 22  kV / 345 kV/LConn3 -- Bus 35/RConn3 -- 5 MW/LConn3
  Machine 6 1000 MVA 22 kV/RConn1 -- Bus 35/LConn1
  Machine 6 1000 MVA 22 kV/RConn2 -- Bus 35/LConn2
  Machine 6 1000 MVA 22 kV/RConn3 -- Bus 35/LConn3
  GT1_CB8/LConn1 -- Transformer 6 880 MVA 22  kV / 345 kV/RConn1
  GT1_CB8/LConn2 -- Transformer 6 880 MVA 22  kV / 345 kV/RConn2
  GT1_CB8/LConn3 -- Transformer 6 880 MVA 22  kV / 345 kV/RConn3
  B/RConn1 -- GT1_CB8/RConn2
  A/RConn1 -- GT1_CB8/RConn1
  C/RConn1 -- GT1_CB8/RConn3

== system model_T_PSH_IEEE39/SS_EastSystem2/GT 7 ==
  5 MW : powerlib/Elements/Three-Phase Parallel RLC Load  LConnTagsString=A|B|C  Configuration=Y (grounded)  NominalVoltage=22e3  Vabc=[1e3 1e3 1e3]  Vabcp=[1e3 1e3 1e3]  NominalFrequency=fNom  UnbalancedPower=off  ActivePower=5e6  InductivePower=0  CapacitivePower=0  Pabc=[10e3 9e3 11e3]  QLabc=[100 90 110]  QCabc=[100 90 110]  Pabcp=[10e3 9e3 11e3]  QLabcp=[100 90 110]  QCabcp=[100 90 110]  Measurements=None  LoadType=constant Z
  Bus Selector1 : BusSelector  OutputSignals="dq0 components.Stator voltage  vq (pu),dq0 components.Stator voltage  vd (pu),Mechanical.Rotor speed  wm  (pu),Mechanical.Rotor speed deviation  dw (pu),Output active power   Peo (pu),Output reactive power  Qeo (pu)"
  Bus 36 : powerlib/Measurements/Three-Phase V-I Measurement  VoltageMeasurement=phase-to-ground  SetLabelV=on  LabelV=V_bus_G7  Vpu=off  VpuLL=off  CurrentMeasurement=no  SetLabelI=on  LabelI=I_bus_G7  Ipu=off  Pbase=100e6  Vbase=16.5e3  OutputType=Complex  PhasorSimulation=off  PSBequivalent=0
  Excitation System : sps_avr/Excitation System  tr=20e-3  reg=[ 200, 0.02 ]  exc=[ 1, 0 .19]  tgr=[ 0, 0 ]  damp=[ 0.0012, 1 ]  sat=[ 0, 0 ]  lim=[ 0, 7.32, 0 ]  v0=[1.015 1.5412]
      settings: SourceProductBaseCode=PS
  GT1_CB10 : Subsystem
  Ground : Ground
  HTG : powerlib/Machines/Hydraulic Turbine and Governor  sm="[ 10/3  0.07 ]"  gate="[  0.01  0.97518  -0.1  0.1 ]"  reg="[  Rp  1.163  0.105  0  0.01  ]"  hyd="[  0  2.67  ]"  dref=0  po=0.42
      settings: SourceProductBaseCode=PS
  Load Flow Bus : powerlib/Measurements/Load Flow Bus  LConnTagsString=a  Phases=single  Connectors=on one side  ID=Bus-36  Vbase=22000  Vref=1.015  Vangle=0  VLF=1.015  VLFb=1  VLFc=1  angleLF=0.3154  angleLFb=0  angleLFc=0
      settings: AttributesFormatString=%<ID>\n%<Vbase>V\n%<VLF>pu\n%<angleLF>deg.
  Machine 7 1000 MVA 22 kV : powerlib/Machines/Synchronous Machine pu Standard  PresetModel=No  MechanicalLoad=Mechanical power Pm  ShowDetailedParameters=on  RotorType=Round  Units=per unit standard parameters  MeasurementBus=off  NominalParameters="[ 1000E6  22000   fNom]"  Reactances1=[ 2.408 0.4 0.2 2.384 1.518 0.2 0.032 ]  Reactances2=[ 0.995, 0.195, 0.155, 0.568, 0.143, 0.16 ]  dAxisTimeConstants=Open-circuit  qAxisTimeConstants=Open-circuit  TimeConstants1=[]  TimeConstants2=[5.66 0.03 1.5 0.04]  TimeConstants3=[]  TimeConstants4=[]  TimeConstants5=[ 9.2, 0.01, 0.01 ]  TimeConstants6=[]  TimeConstants7=[]  TimeConstants8=[]  StatorResistance=0.005  Mechanical=[ 3.23 0.02 20]  PolePairs=20  InitialConditions=[0 -44.8827 0.454166 0.454166 0.454166 -3.41889 -123.419 116.581 1.54123]  SetSaturation=off  Saturation=[0.6404,0.7127,0.8441,0.9214,0.9956,1.082,1.19,1.316,1.457;0.7,0.7698,0.8872,0.9466,0.9969,1.046,1.1,1.151,1.201]  LoadFlowParameters=[1 560000000 23397 0]  TsPowergui=0  TsBlock=-1  IterativeModel=Trapezoidal non iterative  IterativeDiscreteModel=Trapezoidal non iterative  BusType=PV  Pref=4.6e+008  Qref=0  Qmin=-500e6  Qmax=150e6  PLF=0  QLF=0
      settings: AttributesFormatString=\n\n
  Pref : Constant  Value=0.42
  Terminator5 : Terminator
  Transformer 6 880 MVA 22  kV / 345 kV : powerlib/Elements/Three-Phase Transformer (Two Windings)  Winding1Connection=Delta (D1)  Winding2Connection=Yg  CoreType=Three single-phase transformers  SetSaturation=off  Hysteresis=off  DataFile='hysteresis'  SetInitialFlux=off  Measurements=None  UNITS=pu  NominalPower=[ 897.6e6 fNom]  Winding1="[ 22e3  0.0   0.0143*880/100/2]"  Winding2="[ 1.025*345e3 0.0   0.0143*880/100/2]"  Rm=500  Lm=500  L0=0.5  Saturation="[ 0,0  ;  0.005,1.2  ;  1.0,1.4 ]"  InitialFluxes=[ 0.8 , -0.8 , 0.7 ]  BreakLoop=off  DiscreteSolver=Trapezoidal iterative  DataType=off  TransfoNumber=0
  Vref : Constant  Value=1.015
  wref : Constant
  A : PMIOPort  Side=Right
  B : PMIOPort  Port=2  Side=Right
  C : PMIOPort  Port=3  Side=Right
  tag scope: P_G7=global, Q_G7=global, V_G7=global, Wm_G7=global
  wires:
  Ground/1 -> Excitation System/4
  HTG/2 -> Terminator5/1
  Vref/1 -> Excitation System/1
  Pref/1 -> HTG/2
  wref/1 -> HTG/1
  Excitation System/1 -> Machine 7 1000 MVA 22 kV/2
  HTG/1 -> Machine 7 1000 MVA 22 kV/1
  Machine 7 1000 MVA 22 kV/1 -> Bus Selector1/1
  Bus Selector1/1 -> Excitation System/3  "<Stator voltage  vq (pu)>"
  Bus Selector1/2 -> Excitation System/2  "<Stator voltage  vd (pu)>"
  Bus Selector1/3 -> HTG/3, [Wm_G7]  "<Rotor speed  wm  (pu)>"
  Bus Selector1/4 -> HTG/5  "<Rotor speed deviation  dw (pu)>"
  Bus Selector1/5 -> HTG/4, [P_G7]  "<Output active power   Peo (pu)>"
  Bus Selector1/6 -> [Q_G7]  "<Output reactive power  Qeo (pu)>"
  [V_bus_G7] -> [V_G7]
  connections:
  Load Flow Bus/LConn1 -- Transformer 6 880 MVA 22  kV / 345 kV/LConn1 -- Bus 36/RConn1 -- 5 MW/LConn1
  Bus 36/RConn2 -- Transformer 6 880 MVA 22  kV / 345 kV/LConn2 -- 5 MW/LConn2
  Bus 36/RConn3 -- Transformer 6 880 MVA 22  kV / 345 kV/LConn3 -- 5 MW/LConn3
  Machine 7 1000 MVA 22 kV/RConn1 -- Bus 36/LConn1
  Machine 7 1000 MVA 22 kV/RConn2 -- Bus 36/LConn2
  Machine 7 1000 MVA 22 kV/RConn3 -- Bus 36/LConn3
  Transformer 6 880 MVA 22  kV / 345 kV/RConn3 -- GT1_CB10/LConn3
  Transformer 6 880 MVA 22  kV / 345 kV/RConn2 -- GT1_CB10/LConn2
  Transformer 6 880 MVA 22  kV / 345 kV/RConn1 -- GT1_CB10/LConn1
  B/RConn1 -- GT1_CB10/RConn2
  A/RConn1 -- GT1_CB10/RConn1
  C/RConn1 -- GT1_CB10/RConn3

== system model_T_PSH_IEEE39/SS_EastSystem2/Load 21 ==
  Bus_L21 : powerlib/Measurements/Three-Phase V-I Measurement  VoltageMeasurement=phase-to-ground  SetLabelV=off  LabelV=V_Bus_L21  Vpu=off  VpuLL=off  CurrentMeasurement=yes  SetLabelI=on  LabelI=I_L21  Ipu=off  Pbase=100e6  Vbase=230e3  OutputType=Complex  PhasorSimulation=off  PSBequivalent=0
  Terminator : Terminator
  Three-Phase Dynamic Load : powerlib/Elements/Three-Phase Dynamic Load  NominalVoltage=[345e3 fNom]  ActiveReactivePowers=[2.74e+08 1.15e+08]  PositiveSequence=[1.00586 20.5637]  ExternalControl=on  NpNq=[0 0]  TimeConstants="[0  0  0  0]"  MinimumVoltage=0.7  Tfilter=1e-4  LoadFlowParameters=[4,0,0,0,0]
      settings: SourceProductBaseCode=PS
  A : PMIOPort  Side=Left
  B : PMIOPort  Port=2  Side=Left
  C : PMIOPort  Port=3  Side=Left
  tag scope: V_L21=global
  wires:
  Three-Phase Dynamic Load/1 -> Terminator/1
  Bus_L21/1 -> [V_L21]
  [load21] -> Three-Phase Dynamic Load/1
  connections:
  Bus_L21/RConn1 -- Three-Phase Dynamic Load/LConn1
  C/RConn1 -- Bus_L21/LConn3
  B/RConn1 -- Bus_L21/LConn2
  A/RConn1 -- Bus_L21/LConn1
  Bus_L21/RConn2 -- Three-Phase Dynamic Load/LConn2
  Bus_L21/RConn3 -- Three-Phase Dynamic Load/LConn3

== system model_T_PSH_IEEE39/SS_EastSystem2/Load 23 ==
  Bus_L23 : powerlib/Measurements/Three-Phase V-I Measurement  VoltageMeasurement=phase-to-ground  SetLabelV=off  LabelV=V_Bus_L23  Vpu=off  VpuLL=off  CurrentMeasurement=yes  SetLabelI=on  LabelI=I_L23  Ipu=off  Pbase=100e6  Vbase=230e3  OutputType=Complex  PhasorSimulation=off  PSBequivalent=0
  Terminator : Terminator
  Three-Phase Dynamic Load : powerlib/Elements/Three-Phase Dynamic Load  NominalVoltage=[345e3 fNom]  ActiveReactivePowers=[2.475e+08 8.46e+07]  PositiveSequence=[1.0123 23.421]  ExternalControl=on  NpNq=[0 0]  TimeConstants="[0  0  0  0]"  MinimumVoltage=0.7  Tfilter=1e-4  LoadFlowParameters=[4,0,0,0,0]
      settings: SourceProductBaseCode=PS
  A : PMIOPort  Side=Left
  B : PMIOPort  Port=2  Side=Left
  C : PMIOPort  Port=3  Side=Left
  tag scope: V_L23=global
  wires:
  Three-Phase Dynamic Load/1 -> Terminator/1
  Bus_L23/1 -> [V_L23]
  [load23] -> Three-Phase Dynamic Load/1
  connections:
  Three-Phase Dynamic Load/LConn1 -- Bus_L23/RConn1
  C/RConn1 -- Bus_L23/LConn3
  B/RConn1 -- Bus_L23/LConn2
  A/RConn1 -- Bus_L23/LConn1
  Three-Phase Dynamic Load/LConn2 -- Bus_L23/RConn2
  Three-Phase Dynamic Load/LConn3 -- Bus_L23/RConn3

== system model_T_PSH_IEEE39/SS_EastSystem2/Load 24 ==
  Bus_L24 : powerlib/Measurements/Three-Phase V-I Measurement  VoltageMeasurement=phase-to-ground  SetLabelV=off  LabelV=V_Bus_L24  Vpu=off  VpuLL=off  CurrentMeasurement=yes  SetLabelI=on  LabelI=I_L24  Ipu=off  Pbase=100e6  Vbase=230e3  OutputType=Complex  PhasorSimulation=off  PSBequivalent=0
  Terminator : Terminator
  Three-Phase Dynamic Load : powerlib/Elements/Three-Phase Dynamic Load  NominalVoltage=[345e3 fNom]  ActiveReactivePowers=[3.086e+08 -9.2e+07]  PositiveSequence=[1.01137 19.0799]  ExternalControl=on  NpNq=[0 0]  TimeConstants="[0  0  0  0]"  MinimumVoltage=0.7  Tfilter=1e-4  LoadFlowParameters=[4,0,0,0,0]
      settings: SourceProductBaseCode=PS
  A : PMIOPort  Side=Left
  B : PMIOPort  Port=2  Side=Left
  C : PMIOPort  Port=3  Side=Left
  tag scope: V_L24=global
  wires:
  Three-Phase Dynamic Load/1 -> Terminator/1
  Bus_L24/1 -> [V_L24]
  [load24] -> Three-Phase Dynamic Load/1
  connections:
  Three-Phase Dynamic Load/LConn3 -- Bus_L24/RConn3
  Three-Phase Dynamic Load/LConn2 -- Bus_L24/RConn2
  A/RConn1 -- Bus_L24/LConn1
  B/RConn1 -- Bus_L24/LConn2
  C/RConn1 -- Bus_L24/LConn3
  Three-Phase Dynamic Load/LConn1 -- Bus_L24/RConn1

== system model_T_PSH_IEEE39/SS_EastSystem2/Machines Measurements ==
  Mux : Mux  Inputs=2
  Mux3 : Mux
  Mux4 : Mux
  Machines Measurements : Outport
  wires:
  Mux4/1 -> Mux/2
  Mux3/1 -> Mux/1
  [Wm_G7] -> Mux4/4
  [Q_G7] -> Mux4/3
  [P_G7] -> Mux4/2
  [V_G7] -> Mux4/1
  [Wm_G6] -> Mux3/4
  [Q_G6] -> Mux3/3
  [P_G6] -> Mux3/2
  [V_G6] -> Mux3/1
  Mux/1 -> Machines Measurements/1

== system model_T_PSH_IEEE39/SS_NorthSystem1/Buses current_N ==
  Mux3 : Mux
  curremt : Outport
  wires:
  [I_L25] -> Mux3/1
  [I_L26] -> Mux3/2
  [I_L28] -> Mux3/3
  [I_L29] -> Mux3/4
  Mux3/1 -> curremt/1

== system model_T_PSH_IEEE39/SS_NorthSystem1/Buses voltages_N ==
  Mux3 : Mux
  Voltages : Outport
  wires:
  Mux3/1 -> Voltages/1
  [V_L25] -> Mux3/1
  [V_L26] -> Mux3/2
  [V_L28] -> Mux3/3
  [V_L29] -> Mux3/4
